simulink model "Simple_Pendulum_Motion_Simulation"  (R2022b)
settings: Solver=VariableStepAuto  StartTime=0.0  StopTime=10.0  MaxStep=1e-3  RelTol=1e-3
values from neighbouring files (symbols this model uses):
  angular_displacement0 = 5    [Simple_Pendulum_Motion.m]
  g = 9.81    [Simple_Pendulum_Motion.m]    (also in Simple_Pendulum_Motion_Simulation.m)
  L0 = i    [Simple_Pendulum_Motion.m]
libraries: simulink x1
settings Model: Creator=NourAldin  LastModifiedBy=NourAldin

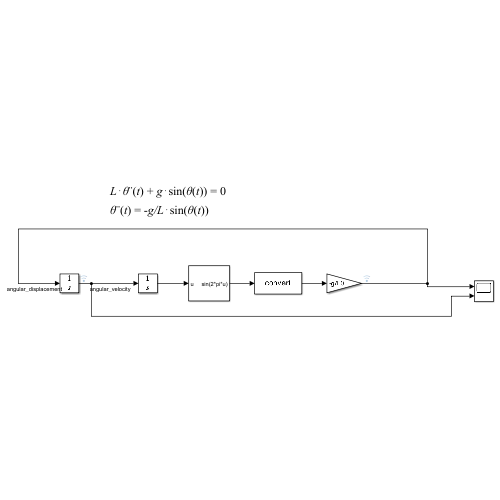
[thumbnail: Simulink's stored preview of the top-level diagram]
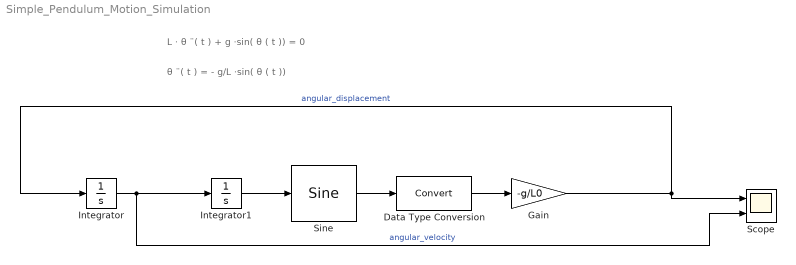
== system Simple_Pendulum_Motion_Simulation ==
  note: L ⋅ θ ¨( t ) + g ⋅sin( θ ( t )) = 0
  note: θ ¨( t ) = - g/L ⋅sin( θ ( t ))
  Data Type Conversion : DataTypeConversion  SaturateOnIntegerOverflow=off  RndMeth=Floor
  Gain : Gain  Gain=-g/L0
  Integrator : Integrator  InitialCondition=angular_displacement0
  Integrator1 : Integrator
  Scope : Scope  NumInputPorts=2
  Sine : simulink/Lookup Tables/Sine  Formula=sin(2*pi*u)  NumDataPoints=(2^5)+1  OutputWordLength=16  InternalRulePriority=Speed
  wires:
  Integrator/1 -> Scope/2, Integrator1/1  "angular_velocity"
  Gain/1 -> Integrator/1, Scope/1  "angular_displacement"
  Integrator1/1 -> Sine/1
  Sine/1 -> Data Type Conversion/1
  Data Type Conversion/1 -> Gain/1
